simulink model "CF016A_GmVehSpdArbn"  (R2013b)
settings: Solver=FixedStepDiscrete  SolverMode=SingleTasking  StartTime=0.0  StopTime=1  FixedStep=0.002  RelTol=1e-3
undefined symbols (not defined in the file): DIAGCSTRTUPDLY_CNT_U32, NODEBSTEP_CNT_U16, NtcNr1, NtcSts1, VEHSPDMAX_KPH_F32
libraries: simulink x8, NxtrMax x7, NxtrMin x3, NxtrLim x3
(part 4 of 5)

== system CF016A_GmVehSpdArbn/GmVehSpdArbn/GmVehSpdArbnPer1/VehSpdMaxSecur_Invld ==
  Action Port : ActionPort  RequirementInfo="{'linktype_rmi_doors' '0000c6e6 (/GM T1XX/SubSystem Specifications/Customer Functions/CF016A GM Vehicle Speed Arbitration)' '#151' 'true' 'REQ:  151' '' } %GIDa_64e2156d_e885_4892_8ce8_3cf277fffe99"  ActionType=then
  Constant3 : Constant  RequirementInfo="{'linktype_rmi_doors' '0000c6e6 (/GM T1XX/SubSystem Specifications/Customer Functions/CF016A GM Vehicle Speed Arbitration)' '#151' 'true' 'REQ:  151' '' } %GIDa_7637d006_42b4_453b_9c6b_38d839e6b7ae"  Value=VEHSPDMAX_KPH_F32  OutDataTypeStr=single
      settings: AttributesFormatString=%<OutDataTypeStr>
  Constant4 : Constant  RequirementInfo="{'linktype_rmi_doors' '0000c6e6 (/GM T1XX/SubSystem Specifications/Customer Functions/CF016A GM Vehicle Speed Arbitration)' '#151' 'true' 'REQ:  151' '' } %GIDa_b234e855_697a_43ff_9746_9b343813ac54"  Value=false  OutDataTypeStr=boolean
      settings: AttributesFormatString=%<OutDataTypeStr>
  CopyRight2 : Subsystem  Description=|  RequirementInfo="{'linktype_rmi_doors' '0000c6e6 (/GM T1XX/SubSystem Specifications/Customer Functions/CF016A GM Vehicle Speed Arbitration)' '#151' 'true' 'REQ:  151' '' } %GIDa_55b8d56c_ea3d_4980_9cc8_0a4d021dc640"  mask(Copyright Information){none=on}
      | Copyright info block.                                               
      |                                                                     
      | Place copyright information at the top of every subsystem in design.
      mask prompts: none "No parameters"
      mask help: Place copyright information at the top of every subsystem in design.
      mask Display:
      | NxtrConf = 'Nexteer Confidential';
      | 
      | sys = bdroot; %handle for the current model ("system")
      | first = get_param(sys,'Created');
      | if(isempty(first))
      |     first = datestr(now,'yyyy');
      | else
      |     first = first(end-3:end);  %year is last four digits
      | end
      | 
      | last = get_param(sys,'LastModifiedDate');
      | if isempty(last)
      |     last = datestr(now,'yyyy');
      | else
      |     last = last(end-3:end);
      | end
      | 
      | if strcmp(first,last)
      |     fprintf('%s -- Copyright %s Nexteer',NxtrConf,first)
      | else
      |     fprintf('%s -- %s%s- %s Nexteer',NxtrConf,char(169),first,last)
      | end
  VehSpdMaxSecur : Outport  RequirementInfo="{'linktype_rmi_doors' '0000c6e6 (/GM T1XX/SubSystem Specifications/Customer Functions/CF016A GM Vehicle Speed Arbitration)' '#151' 'true' 'REQ:  151' '' } %GIDa_f81d9856_2c99_43a9_8580_21441ed5cbe9"
  VehSpdMaxSecurVld : Outport  RequirementInfo="{'linktype_rmi_doors' '0000c6e6 (/GM T1XX/SubSystem Specifications/Customer Functions/CF016A GM Vehicle Speed Arbitration)' '#151' 'true' 'REQ:  151' '' } %GIDa_72ce18ea_7958_4c7d_99d9_9239c29e1241"  Port=2
  wires:
  Constant3/1 -> VehSpdMaxSecur/1
  Constant4/1 -> VehSpdMaxSecurVld/1

== system CF016A_GmVehSpdArbn/GmVehSpdArbn/GmVehSpdArbnPer1/VehSpdMinSecur_Invld ==
  Action Port : ActionPort  ActionType=then
  Constant2 : Constant  RequirementInfo="{'linktype_rmi_doors' '0000c6e6 (/GM T1XX/SubSystem Specifications/Customer Functions/CF016A GM Vehicle Speed Arbitration)' '#200' 'true' 'REQ:  200' '' } %GIDa_8379dec2_765f_4e7e_be43_ecf0c6a82445"  Value=false  OutDataTypeStr=boolean
      settings: AttributesFormatString=%<OutDataTypeStr>
  Constant3 : Constant  RequirementInfo="{'linktype_rmi_doors' '0000c6e6 (/GM T1XX/SubSystem Specifications/Customer Functions/CF016A GM Vehicle Speed Arbitration)' '#200' 'true' 'REQ:  200' '' } %GIDa_805cec81_7588_4ea2_95e1_c6a565f2085e"  Value=0  OutDataTypeStr=single
      settings: AttributesFormatString=%<OutDataTypeStr>
  CopyRight2 : Subsystem  Description=|  mask(Copyright Information){none=on}
      | Copyright info block.                                               
      |                                                                     
      | Place copyright information at the top of every subsystem in design.
      mask prompts: none "No parameters"
      mask help: Place copyright information at the top of every subsystem in design.
      mask Display:
      | NxtrConf = 'Nexteer Confidential';
      | 
      | sys = bdroot; %handle for the current model ("system")
      | first = get_param(sys,'Created');
      | if(isempty(first))
      |     first = datestr(now,'yyyy');
      | else
      |     first = first(end-3:end);  %year is last four digits
      | end
      | 
      | last = get_param(sys,'LastModifiedDate');
      | if isempty(last)
      |     last = datestr(now,'yyyy');
      | else
      |     last = last(end-3:end);
      | end
      | 
      | if strcmp(first,last)
      |     fprintf('%s -- Copyright %s Nexteer',NxtrConf,first)
      | else
      |     fprintf('%s -- %s%s- %s Nexteer',NxtrConf,char(169),first,last)
      | end
  VehSpdMinSecur : Outport  RequirementInfo="{'linktype_rmi_doors' '0000c6e6 (/GM T1XX/SubSystem Specifications/Customer Functions/CF016A GM Vehicle Speed Arbitration)' '#200' 'true' 'REQ:  200' '' } %GIDa_4848a70f_3ce8_4b37_84fd_cdad733c9f51"
  VehSpdMinSecurVld : Outport  RequirementInfo="{'linktype_rmi_doors' '0000c6e6 (/GM T1XX/SubSystem Specifications/Customer Functions/CF016A GM Vehicle Speed Arbitration)' '#200' 'true' 'REQ:  200' '' } %GIDa_aef7dbb3_b6b0_484d_bb99_ef1c2a4a1cac"  Port=2
  wires:
  Constant2/1 -> VehSpdMinSecurVld/1
  Constant3/1 -> VehSpdMinSecur/1

== system CF016A_GmVehSpdArbn/GmVehSpdArbn/GmVehSpdArbnInit1/GetRefTmr100MicroSec32bit/CopyRight2 ==

== system CF016A_GmVehSpdArbn/GmVehSpdArbn/GmVehSpdArbnPer1/ArbdFalseAndSnsrFalse_NTCFaild/CopyRight2 ==

== system CF016A_GmVehSpdArbn/GmVehSpdArbn/GmVehSpdArbnPer1/ArbdFalseAndSnsrFalse_NTCFaild/NTC_0x0E0 ==
  NtcNr : Inport
  NtcStInfo : Inport  Port=2
  NtcSts : Inport  Port=3
  DebStep : Inport  Port=4
  CallDiagMgr : ActionPort  ActionType=then
  SetNtcSts : Subsystem  RequirementInfo={} %GIDa_9ed89afc_c0fd_408c_a804_1b2e1348b82a  TreatAsAtomicUnit=on
      settings: RTWSystemCode=Inline
  wires:
  NtcNr/1 -> SetNtcSts/1(NtcNr)  "NtcNr"
  NtcSts/1 -> SetNtcSts/3(NtcSts)
  DebStep/1 -> SetNtcSts/4(DebStep)
  NtcStInfo/1 -> SetNtcSts/2(NtcStInfo)

== system CF016A_GmVehSpdArbn/GmVehSpdArbn/GmVehSpdArbnPer1/ArbdFalseAndSnsrTrue_NTCPassd/CopyRight2 ==

== system CF016A_GmVehSpdArbn/GmVehSpdArbn/GmVehSpdArbnPer1/ArbdFalseAndSnsrTrue_NTCPassd/NTC_0x0E0 ==
  NtcNr : Inport
  NtcStInfo : Inport  Port=2
  NtcSts : Inport  Port=3
  DebStep : Inport  Port=4
  CallDiagMgr : ActionPort  ActionType=then
  SetNtcSts : Subsystem  RequirementInfo={} %GIDa_edd408d1_9bb5_4017_8804_a8b180852b3e  TreatAsAtomicUnit=on
      settings: RTWSystemCode=Inline
  wires:
  NtcStInfo/1 -> SetNtcSts/2(NtcStInfo)
  DebStep/1 -> SetNtcSts/4(DebStep)
  NtcSts/1 -> SetNtcSts/3(NtcSts)
  NtcNr/1 -> SetNtcSts/1(NtcNr)  "NtcNr"

== system CF016A_GmVehSpdArbn/GmVehSpdArbn/GmVehSpdArbnPer1/ArbdTrueAndSnsrTrue_NTCPassd/CopyRight2 ==

== system CF016A_GmVehSpdArbn/GmVehSpdArbn/GmVehSpdArbnPer1/ArbdTrueAndSnsrTrue_NTCPassd/NTC_0x0E0 ==
  NtcNr : Inport
  NtcStInfo : Inport  Port=2
  NtcSts : Inport  Port=3
  DebStep : Inport  Port=4
  CallDiagMgr : ActionPort  ActionType=then
  SetNtcSts : Subsystem  RequirementInfo={} %GIDa_c0105d74_7713_458a_af4f_14b36b448539  TreatAsAtomicUnit=on
      settings: RTWSystemCode=Inline
  wires:
  NtcStInfo/1 -> SetNtcSts/2(NtcStInfo)
  DebStep/1 -> SetNtcSts/4(DebStep)
  NtcSts/1 -> SetNtcSts/3(NtcSts)
  NtcNr/1 -> SetNtcSts/1(NtcNr)  "NtcNr"

== system CF016A_GmVehSpdArbn/GmVehSpdArbn/GmVehSpdArbnPer1/Calc_NTCIdleTi/CopyRight2 ==

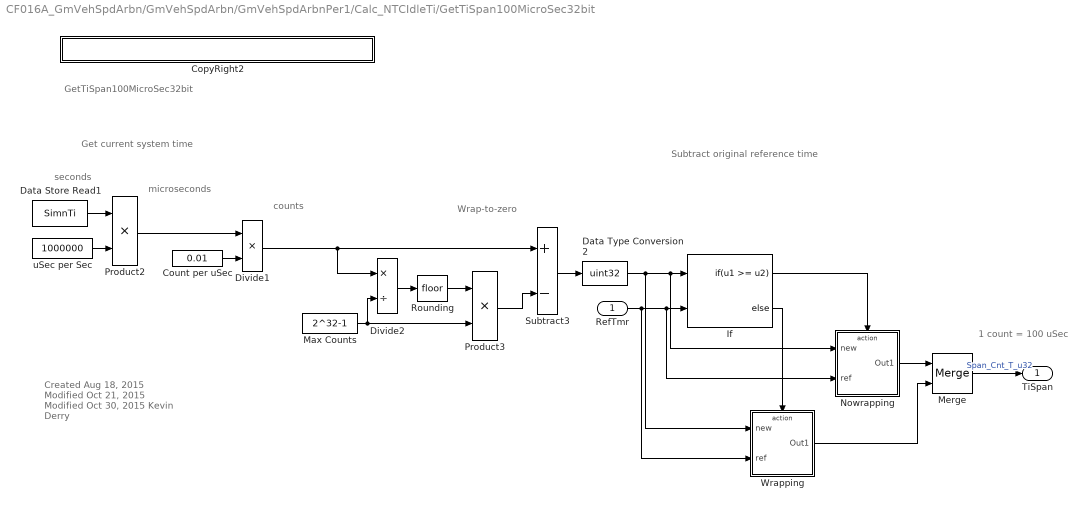
== system CF016A_GmVehSpdArbn/GmVehSpdArbn/GmVehSpdArbnPer1/Calc_NTCIdleTi/GetTiSpan100MicroSec32bit ==
  note: Created Aug 18, 2015
      | Modified Oct 21, 2015
      | Modified Oct 30, 2015
      | Kevin Derry
  note: GetTiSpan100MicroSec32bit
  note: Get current system time
  note: 1 count = 100 uSec
  note: Wrap-to-zero
  note: counts
  note: microseconds
  note: seconds
  note: Subtract original reference time
  RefTmr : Inport
  CopyRight2 : Subsystem  Description=|  mask(Copyright Information){none=on}
      | Copyright info block.                                               
      |                                                                     
      | Place copyright information at the top of every subsystem in design.
      mask prompts: none "No parameters"
      mask help: Place copyright information at the top of every subsystem in design.
      mask Display:
      | NxtrConf = 'Nexteer Confidential';
      | 
      | sys = bdroot; %handle for the current model ("system")
      | first = get_param(sys,'Created');
      | if(isempty(first))
      |     first = datestr(now,'yyyy');
      | else
      |     first = first(end-3:end);  %year is last four digits
      | end
      | 
      | last = get_param(sys,'LastModifiedDate');
      | if isempty(last)
      |     last = datestr(now,'yyyy');
      | else
      |     last = last(end-3:end);
      | end
      | 
      | if strcmp(first,last)
      |     fprintf('%s -- Copyright %s Nexteer',NxtrConf,first)
      | else
      |     fprintf('%s -- %s%s- %s Nexteer',NxtrConf,char(169),first,last)
      | end
  Count per uSec : Constant  Value=0.01
  Data Store Read1 : DataStoreRead  DataStoreName=SimnTi
  Data Type Conversion2 : DataTypeConversion  OutDataTypeStr=uint32
  Divide1 : Product  Inputs=**
  Divide2 : Product  Inputs=*/
  If : If  NumInputs=2  IfExpression=u1 >= u2
  Max Counts : Constant  Value=2^32-1
  Merge : Merge
  Nowrapping : Subsystem  TreatAsAtomicUnit=on
  Product2 : Product
  Product3 : Product
  Rounding : Rounding
  Subtract3 : Sum  Inputs=+-
  Wrapping : Subsystem  TreatAsAtomicUnit=on
  uSec per Sec : Constant  Value=1000000
  TiSpan : Outport
  wires:
  Data Type Conversion2/1 -> Wrapping/1(new), Nowrapping/1(new), If/1
  RefTmr/1 -> Wrapping/2(ref), Nowrapping/2(ref), If/2
  Merge/1 -> TiSpan/1  "Span_Cnt_T_u32"
  uSec per Sec/1 -> Product2/2
  Count per uSec/1 -> Divide1/2
  Data Store Read1/1 -> Product2/1
  Product2/1 -> Divide1/1
  Divide1/1 -> Subtract3/1, Divide2/1
  Max Counts/1 -> Product3/2, Divide2/2
  Divide2/1 -> Rounding/1
  Rounding/1 -> Product3/1
  Subtract3/1 -> Data Type Conversion2/1
  Product3/1 -> Subtract3/2
  If/1 -> Nowrapping/Action
  If/2 -> Wrapping/Action
  Nowrapping/1(Out1) -> Merge/1
  Wrapping/1(Out1) -> Merge/2

== system CF016A_GmVehSpdArbn/GmVehSpdArbn/GmVehSpdArbnPer1/Calc_SpdArbd/Calc_VehSpdArbd ==
  TmpSpdArbd : Inport  RequirementInfo={} %GIDa_22ee0604_b96b_41df_b3cf_508af8afbd88
  TmpSpdArbdCnt : Inport  RequirementInfo={} %GIDa_d3815bce_edc7_4bfa_b1ce_5bf581d265aa  Port=2
  Action Port : ActionPort  ActionType=then
  CopyRight2 : Subsystem  Description=|  mask(Copyright Information){none=on}
      | Copyright info block.                                               
      |                                                                     
      | Place copyright information at the top of every subsystem in design.
      mask prompts: none "No parameters"
      mask help: Place copyright information at the top of every subsystem in design.
      mask Display:
      | NxtrConf = 'Nexteer Confidential';
      | 
      | sys = bdroot; %handle for the current model ("system")
      | first = get_param(sys,'Created');
      | if(isempty(first))
      |     first = datestr(now,'yyyy');
      | else
      |     first = first(end-3:end);  %year is last four digits
      | end
      | 
      | last = get_param(sys,'LastModifiedDate');
      | if isempty(last)
      |     last = datestr(now,'yyyy');
      | else
      |     last = last(end-3:end);
      | end
      | 
      | if strcmp(first,last)
      |     fprintf('%s -- Copyright %s Nexteer',NxtrConf,first)
      | else
      |     fprintf('%s -- %s%s- %s Nexteer',NxtrConf,char(169),first,last)
      | end
  Divide : Product  Inputs=*/
  SpdArbd : Outport
  wires:
  TmpSpdArbd/1 -> Divide/1
  TmpSpdArbdCnt/1 -> Divide/2
  Divide/1 -> SpdArbd/1

== system CF016A_GmVehSpdArbn/GmVehSpdArbn/GmVehSpdArbnPer1/Calc_SpdArbd/CopyRight2 ==

== system CF016A_GmVehSpdArbn/GmVehSpdArbn/GmVehSpdArbnPer1/Calc_SpdArbd/Pass_TmpSpdArbd ==
  TmpSpdArbd : Inport  RequirementInfo={} %GIDa_a9ccc6d1_62c5_46ea_817b_212a243cba27
  Action Port : ActionPort  ActionType=else
  CopyRight2 : Subsystem  Description=|  mask(Copyright Information){none=on}
      | Copyright info block.                                               
      |                                                                     
      | Place copyright information at the top of every subsystem in design.
      mask prompts: none "No parameters"
      mask help: Place copyright information at the top of every subsystem in design.
      mask Display:
      | NxtrConf = 'Nexteer Confidential';
      | 
      | sys = bdroot; %handle for the current model ("system")
      | first = get_param(sys,'Created');
      | if(isempty(first))
      |     first = datestr(now,'yyyy');
      | else
      |     first = first(end-3:end);  %year is last four digits
      | end
      | 
      | last = get_param(sys,'LastModifiedDate');
      | if isempty(last)
      |     last = datestr(now,'yyyy');
      | else
      |     last = last(end-3:end);
      | end
      | 
      | if strcmp(first,last)
      |     fprintf('%s -- Copyright %s Nexteer',NxtrConf,first)
      | else
      |     fprintf('%s -- %s%s- %s Nexteer',NxtrConf,char(169),first,last)
      | end
  VehSpdArbd : Outport
  wires:
  TmpSpdArbd/1 -> VehSpdArbd/1

== system CF016A_GmVehSpdArbn/GmVehSpdArbn/GmVehSpdArbnPer1/Calc_TmpSpdArbd_SpdArbdCnt/CalcSumCnt ==
  TmpSpdIn : Inport  RequirementInfo={} %GIDa_cc3fdd2f_e00a_4d73_ad47_b131220ca799
  RiDrvnBusHiSpd : Inport  RequirementInfo={} %GIDa_bdf168f4_a9f1_4976_b82a_f5282d73e040  Port=2
  CntIn : Inport  RequirementInfo={} %GIDa_335889c6_d315_49b5_8e0c_287140eef7c6  Port=3
  Action Port : ActionPort  ActionType=then
  Add : Sum
  Add1 : Sum
  Constant2 : Constant  OutDataTypeStr=single
      settings: AttributesFormatString=%<OutDataTypeStr>
  CopyRight2 : Subsystem  Description=|  mask(Copyright Information){none=on}
      | Copyright info block.                                               
      |                                                                     
      | Place copyright information at the top of every subsystem in design.
      mask prompts: none "No parameters"
      mask help: Place copyright information at the top of every subsystem in design.
      mask Display:
      | NxtrConf = 'Nexteer Confidential';
      | 
      | sys = bdroot; %handle for the current model ("system")
      | first = get_param(sys,'Created');
      | if(isempty(first))
      |     first = datestr(now,'yyyy');
      | else
      |     first = first(end-3:end);  %year is last four digits
      | end
      | 
      | last = get_param(sys,'LastModifiedDate');
      | if isempty(last)
      |     last = datestr(now,'yyyy');
      | else
      |     last = last(end-3:end);
      | end
      | 
      | if strcmp(first,last)
      |     fprintf('%s -- Copyright %s Nexteer',NxtrConf,first)
      | else
      |     fprintf('%s -- %s%s- %s Nexteer',NxtrConf,char(169),first,last)
      | end
  TmpSpdArbd : Outport
  SpdArbdCnt : Outport  Port=2
  wires:
  Add1/1 -> SpdArbdCnt/1
  Constant2/1 -> Add1/2
  CntIn/1 -> Add1/1
  TmpSpdIn/1 -> Add/2
  RiDrvnBusHiSpd/1 -> Add/1
  Add/1 -> TmpSpdArbd/1

== system CF016A_GmVehSpdArbn/GmVehSpdArbn/GmVehSpdArbnPer1/Calc_TmpSpdArbd_SpdArbdCnt/CalcSumCnt_1 ==
  LeNonDrvnBusHiSpd : Inport  RequirementInfo={} %GIDa_850f1153_ec6b_472c_bf3f_b4555508d628
  TmpSpdIn : Inport  RequirementInfo={} %GIDa_8bdfcdcf_300c_498e_8ae0_3709bc028ab2  Port=2
  CntIn : Inport  RequirementInfo={} %GIDa_524e2e91_4b78_4f70_98dc_26836a52cb3a  Port=3
  Action Port : ActionPort  ActionType=then
  Add : Sum
  Add1 : Sum
  Constant2 : Constant  OutDataTypeStr=single
      settings: AttributesFormatString=%<OutDataTypeStr>
  CopyRight2 : Subsystem  Description=|  mask(Copyright Information){none=on}
      | Copyright info block.                                               
      |                                                                     
      | Place copyright information at the top of every subsystem in design.
      mask prompts: none "No parameters"
      mask help: Place copyright information at the top of every subsystem in design.
      mask Display:
      | NxtrConf = 'Nexteer Confidential';
      | 
      | sys = bdroot; %handle for the current model ("system")
      | first = get_param(sys,'Created');
      | if(isempty(first))
      |     first = datestr(now,'yyyy');
      | else
      |     first = first(end-3:end);  %year is last four digits
      | end
      | 
      | last = get_param(sys,'LastModifiedDate');
      | if isempty(last)
      |     last = datestr(now,'yyyy');
      | else
      |     last = last(end-3:end);
      | end
      | 
      | if strcmp(first,last)
      |     fprintf('%s -- Copyright %s Nexteer',NxtrConf,first)
      | else
      |     fprintf('%s -- %s%s- %s Nexteer',NxtrConf,char(169),first,last)
      | end
  TmpSpdArbd : Outport
  SpdArbdCnt : Outport  Port=2
  wires:
  Add/1 -> TmpSpdArbd/1
  TmpSpdIn/1 -> Add/1
  LeNonDrvnBusHiSpd/1 -> Add/2
  CntIn/1 -> Add1/1
  Constant2/1 -> Add1/2
  Add1/1 -> SpdArbdCnt/1

== system CF016A_GmVehSpdArbn/GmVehSpdArbn/GmVehSpdArbnPer1/Calc_TmpSpdArbd_SpdArbdCnt/CalcSumCnt_2 ==
  TmpSpdIn : Inport  RequirementInfo={} %GIDa_8e0c55ff_68c1_41a4_a413_79990270a578
  RiNonDrvnBusHiSpd : Inport  RequirementInfo={} %GIDa_75592bc1_7625_4699_8c9b_f1eb2e030f50  Port=2
  CntIn : Inport  RequirementInfo={} %GIDa_c479272c_0732_4e1a_8e5e_d31eed4afd4e  Port=3
  Action Port : ActionPort  ActionType=then
  Add : Sum
  Add1 : Sum
  Constant2 : Constant  OutDataTypeStr=single
      settings: AttributesFormatString=%<OutDataTypeStr>
  CopyRight2 : Subsystem  Description=|  mask(Copyright Information){none=on}
      | Copyright info block.                                               
      |                                                                     
      | Place copyright information at the top of every subsystem in design.
      mask prompts: none "No parameters"
      mask help: Place copyright information at the top of every subsystem in design.
      mask Display:
      | NxtrConf = 'Nexteer Confidential';
      | 
      | sys = bdroot; %handle for the current model ("system")
      | first = get_param(sys,'Created');
      | if(isempty(first))
      |     first = datestr(now,'yyyy');
      | else
      |     first = first(end-3:end);  %year is last four digits
      | end
      | 
      | last = get_param(sys,'LastModifiedDate');
      | if isempty(last)
      |     last = datestr(now,'yyyy');
      | else
      |     last = last(end-3:end);
      | end
      | 
      | if strcmp(first,last)
      |     fprintf('%s -- Copyright %s Nexteer',NxtrConf,first)
      | else
      |     fprintf('%s -- %s%s- %s Nexteer',NxtrConf,char(169),first,last)
      | end
  TmpSpdArbd : Outport
  SpdArbdCnt : Outport  Port=2
  wires:
  Add1/1 -> SpdArbdCnt/1
  Constant2/1 -> Add1/2
  CntIn/1 -> Add1/1
  TmpSpdIn/1 -> Add/2
  RiNonDrvnBusHiSpd/1 -> Add/1
  Add/1 -> TmpSpdArbd/1

== system CF016A_GmVehSpdArbn/GmVehSpdArbn/GmVehSpdArbnPer1/Calc_TmpSpdArbd_SpdArbdCnt/CalcSumCnt_3 ==
  TmpSpdIn : Inport  RequirementInfo={} %GIDa_27ed8032_b8a3_44e7_a82c_716af4549a85
  LeDrvnBusHiSpd : Inport  RequirementInfo={} %GIDa_c96c6b2e_7259_40ac_8462_8989bfe94a44  Port=2
  CntIn : Inport  RequirementInfo={} %GIDa_dfbf4464_a6c1_42ad_8ec2_154e9928d5a6  Port=3
  Action Port : ActionPort  ActionType=then
  Add : Sum
  Add1 : Sum
  Constant2 : Constant  OutDataTypeStr=single
      settings: AttributesFormatString=%<OutDataTypeStr>
  CopyRight2 : Subsystem  Description=|  mask(Copyright Information){none=on}
      | Copyright info block.                                               
      |                                                                     
      | Place copyright information at the top of every subsystem in design.
      mask prompts: none "No parameters"
      mask help: Place copyright information at the top of every subsystem in design.
      mask Display:
      | NxtrConf = 'Nexteer Confidential';
      | 
      | sys = bdroot; %handle for the current model ("system")
      | first = get_param(sys,'Created');
      | if(isempty(first))
      |     first = datestr(now,'yyyy');
      | else
      |     first = first(end-3:end);  %year is last four digits
      | end
      | 
      | last = get_param(sys,'LastModifiedDate');
      | if isempty(last)
      |     last = datestr(now,'yyyy');
      | else
      |     last = last(end-3:end);
      | end
      | 
      | if strcmp(first,last)
      |     fprintf('%s -- Copyright %s Nexteer',NxtrConf,first)
      | else
      |     fprintf('%s -- %s%s- %s Nexteer',NxtrConf,char(169),first,last)
      | end
  TmpSpdArbd : Outport
  SpdArbdCnt : Outport  Port=2
  wires:
  Add/1 -> TmpSpdArbd/1
  LeDrvnBusHiSpd/1 -> Add/1
  TmpSpdIn/1 -> Add/2
  CntIn/1 -> Add1/1
  Constant2/1 -> Add1/2
  Add1/1 -> SpdArbdCnt/1

== system CF016A_GmVehSpdArbn/GmVehSpdArbn/GmVehSpdArbnPer1/Calc_TmpSpdArbd_SpdArbdCnt/CopyRight2 ==

== system CF016A_GmVehSpdArbn/GmVehSpdArbn/GmVehSpdArbnPer1/Calc_TmpSpdArbd_SpdArbdCnt/Pass_0s ==
  TmpSpdIn : Inport  RequirementInfo={} %GIDa_c245ec3d_ac7f_433e_a7eb_117742686023
  CntIn : Inport  RequirementInfo={} %GIDa_04336cb5_f5d6_482b_a7a3_24a26aa66881  Port=2
  Action Port : ActionPort  ActionType=else
  CopyRight2 : Subsystem  Description=|  mask(Copyright Information){none=on}
      | Copyright info block.                                               
      |                                                                     
      | Place copyright information at the top of every subsystem in design.
      mask prompts: none "No parameters"
      mask help: Place copyright information at the top of every subsystem in design.
      mask Display:
      | NxtrConf = 'Nexteer Confidential';
      | 
      | sys = bdroot; %handle for the current model ("system")
      | first = get_param(sys,'Created');
      | if(isempty(first))
      |     first = datestr(now,'yyyy');
      | else
      |     first = first(end-3:end);  %year is last four digits
      | end
      | 
      | last = get_param(sys,'LastModifiedDate');
      | if isempty(last)
      |     last = datestr(now,'yyyy');
      | else
      |     last = last(end-3:end);
      | end
      | 
      | if strcmp(first,last)
      |     fprintf('%s -- Copyright %s Nexteer',NxtrConf,first)
      | else
      |     fprintf('%s -- %s%s- %s Nexteer',NxtrConf,char(169),first,last)
      | end
  TmpSpdArbd : Outport
  SpdArbdCnt : Outport  Port=2
  wires:
  CntIn/1 -> SpdArbdCnt/1
  TmpSpdIn/1 -> TmpSpdArbd/1

== system CF016A_GmVehSpdArbn/GmVehSpdArbn/GmVehSpdArbnPer1/Calc_TmpSpdArbd_SpdArbdCnt/Pass_TmpSpdArbd_SpdArbdCnt_1 ==
  TmpSpdIn : Inport  RequirementInfo={} %GIDa_be392035_672d_4555_8348_f6cb397ff1c2
  CntIn : Inport  RequirementInfo={} %GIDa_b54fbdf8_af01_4bd7_a959_8ca2986c3520  Port=2
  Action Port : ActionPort  ActionType=else
  CopyRight2 : Subsystem  Description=|  mask(Copyright Information){none=on}
      | Copyright info block.                                               
      |                                                                     
      | Place copyright information at the top of every subsystem in design.
      mask prompts: none "No parameters"
      mask help: Place copyright information at the top of every subsystem in design.
      mask Display:
      | NxtrConf = 'Nexteer Confidential';
      | 
      | sys = bdroot; %handle for the current model ("system")
      | first = get_param(sys,'Created');
      | if(isempty(first))
      |     first = datestr(now,'yyyy');
      | else
      |     first = first(end-3:end);  %year is last four digits
      | end
      | 
      | last = get_param(sys,'LastModifiedDate');
      | if isempty(last)
      |     last = datestr(now,'yyyy');
      | else
      |     last = last(end-3:end);
      | end
      | 
      | if strcmp(first,last)
      |     fprintf('%s -- Copyright %s Nexteer',NxtrConf,first)
      | else
      |     fprintf('%s -- %s%s- %s Nexteer',NxtrConf,char(169),first,last)
      | end
  TmpSpdArbd : Outport
  SpdArbdCnt : Outport  Port=2
  wires:
  CntIn/1 -> SpdArbdCnt/1
  TmpSpdIn/1 -> TmpSpdArbd/1

== system CF016A_GmVehSpdArbn/GmVehSpdArbn/GmVehSpdArbnPer1/Calc_TmpSpdArbd_SpdArbdCnt/Pass_TmpSpdArbd_SpdArbdCnt_2 ==
  TmpSpdIn : Inport  RequirementInfo={} %GIDa_c2285e44_32b2_4691_a335_e8a509434fe3
  CntIn : Inport  RequirementInfo={} %GIDa_b6863996_5c43_4ec4_8339_06ddcee963ca  Port=2
  Action Port : ActionPort  ActionType=else
  CopyRight2 : Subsystem  Description=|  mask(Copyright Information){none=on}
      | Copyright info block.                                               
      |                                                                     
      | Place copyright information at the top of every subsystem in design.
      mask prompts: none "No parameters"
      mask help: Place copyright information at the top of every subsystem in design.
      mask Display:
      | NxtrConf = 'Nexteer Confidential';
      | 
      | sys = bdroot; %handle for the current model ("system")
      | first = get_param(sys,'Created');
      | if(isempty(first))
      |     first = datestr(now,'yyyy');
      | else
      |     first = first(end-3:end);  %year is last four digits
      | end
      | 
      | last = get_param(sys,'LastModifiedDate');
      | if isempty(last)
      |     last = datestr(now,'yyyy');
      | else
      |     last = last(end-3:end);
      | end
      | 
      | if strcmp(first,last)
      |     fprintf('%s -- Copyright %s Nexteer',NxtrConf,first)
      | else
      |     fprintf('%s -- %s%s- %s Nexteer',NxtrConf,char(169),first,last)
      | end
  TmpSpdArbd : Outport
  SpdArbdCnt : Outport  Port=2
  wires:
  TmpSpdIn/1 -> TmpSpdArbd/1
  CntIn/1 -> SpdArbdCnt/1

== system CF016A_GmVehSpdArbn/GmVehSpdArbn/GmVehSpdArbnPer1/Calc_TmpSpdArbd_SpdArbdCnt/Pass_TmpSpdArbd_SpdArbdCnt_3 ==
  TmpSpdIn : Inport  RequirementInfo={} %GIDa_5e5df1f6_8ff4_4858_9989_4bafd778ca0f
  CntIn : Inport  RequirementInfo={} %GIDa_0592b7e3_be9b_4836_9a53_c8b365bd076c  Port=2
  Action Port : ActionPort  ActionType=else
  CopyRight2 : Subsystem  Description=|  mask(Copyright Information){none=on}
      | Copyright info block.                                               
      |                                                                     
      | Place copyright information at the top of every subsystem in design.
      mask prompts: none "No parameters"
      mask help: Place copyright information at the top of every subsystem in design.
      mask Display:
      | NxtrConf = 'Nexteer Confidential';
      | 
      | sys = bdroot; %handle for the current model ("system")
      | first = get_param(sys,'Created');
      | if(isempty(first))
      |     first = datestr(now,'yyyy');
      | else
      |     first = first(end-3:end);  %year is last four digits
      | end
      | 
      | last = get_param(sys,'LastModifiedDate');
      | if isempty(last)
      |     last = datestr(now,'yyyy');
      | else
      |     last = last(end-3:end);
      | end
      | 
      | if strcmp(first,last)
      |     fprintf('%s -- Copyright %s Nexteer',NxtrConf,first)
      | else
      |     fprintf('%s -- %s%s- %s Nexteer',NxtrConf,char(169),first,last)
      | end
  TmpSpdArbd : Outport
  SpdArbdCnt : Outport  Port=2
  wires:
  CntIn/1 -> SpdArbdCnt/1
  TmpSpdIn/1 -> TmpSpdArbd/1

== system CF016A_GmVehSpdArbn/GmVehSpdArbn/GmVehSpdArbnPer1/Calc_VehSpdMaxSecur/Calc_VehSpdMaxSecur ==
  VehSpdMaxSecur : Inport  RequirementInfo={} %GIDa_b1037a0f_d275_40dd_a845_e9fde032183c
  WhlGndVelRiNonDrvnBusChassisExp : Inport  RequirementInfo={} %GIDa_398e957f_9e7e_45fc_917b_0fc3d04e1e46  Port=2
  WhlGndVelRiNonDrvnBusHiSpd : Inport  RequirementInfo={} %GIDa_085660d0_509a_4113_872b_79769319dc23  Port=3
  Action Port : ActionPort  ActionType=then
  CopyRight2 : Subsystem  Description=|  mask(Copyright Information){none=on}
      | Copyright info block.                                               
      |                                                                     
      | Place copyright information at the top of every subsystem in design.
      mask prompts: none "No parameters"
      mask help: Place copyright information at the top of every subsystem in design.
      mask Display:
      | NxtrConf = 'Nexteer Confidential';
      | 
      | sys = bdroot; %handle for the current model ("system")
      | first = get_param(sys,'Created');
      | if(isempty(first))
      |     first = datestr(now,'yyyy');
      | else
      |     first = first(end-3:end);  %year is last four digits
      | end
      | 
      | last = get_param(sys,'LastModifiedDate');
      | if isempty(last)
      |     last = datestr(now,'yyyy');
      | else
      |     last = last(end-3:end);
      | end
      | 
      | if strcmp(first,last)
      |     fprintf('%s -- Copyright %s Nexteer',NxtrConf,first)
      | else
      |     fprintf('%s -- %s%s- %s Nexteer',NxtrConf,char(169),first,last)
      | end
  Max_f1 : NxtrMax/Max_f32  SFunctionSpec=single y1 = Max_f32(single u1, single u2)
      settings: AttributesFormatString=%<Name>
  Max_f32 : NxtrMax/Max_f32  SFunctionSpec=single y1 = Max_f32(single u1, single u2)
      settings: AttributesFormatString=%<Name>
  TmpVehSpdMaxSecur : Outport
  wires:
  Max_f1/1 -> TmpVehSpdMaxSecur/1
  Max_f32/1 -> Max_f1/1
  VehSpdMaxSecur/1 -> Max_f32/1
  WhlGndVelRiNonDrvnBusChassisExp/1 -> Max_f32/2
  WhlGndVelRiNonDrvnBusHiSpd/1 -> Max_f1/2

== system CF016A_GmVehSpdArbn/GmVehSpdArbn/GmVehSpdArbnPer1/Calc_VehSpdMaxSecur/Calc_VehSpdMaxSecur1 ==
  WhlGndVelLeDrvnBusChassisExp : Inport  RequirementInfo={} %GIDa_a5714172_ef06_41ef_b8c5_c003cd29fe6a  OutDataTypeStr=single
  WhlGndVelLeDrvnBusHiSpd : Inport  RequirementInfo={} %GIDa_0d911216_cd59_4389_bf95_6fb3bce5f572  Port=2
  Action Port : ActionPort  ActionType=then
  CopyRight2 : Subsystem  Description=|  mask(Copyright Information){none=on}
      | Copyright info block.                                               
      |                                                                     
      | Place copyright information at the top of every subsystem in design.
      mask prompts: none "No parameters"
      mask help: Place copyright information at the top of every subsystem in design.
      mask Display:
      | NxtrConf = 'Nexteer Confidential';
      | 
      | sys = bdroot; %handle for the current model ("system")
      | first = get_param(sys,'Created');
      | if(isempty(first))
      |     first = datestr(now,'yyyy');
      | else
      |     first = first(end-3:end);  %year is last four digits
      | end
      | 
      | last = get_param(sys,'LastModifiedDate');
      | if isempty(last)
      |     last = datestr(now,'yyyy');
      | else
      |     last = last(end-3:end);
      | end
      | 
      | if strcmp(first,last)
      |     fprintf('%s -- Copyright %s Nexteer',NxtrConf,first)
      | else
      |     fprintf('%s -- %s%s- %s Nexteer',NxtrConf,char(169),first,last)
      | end
  Max_f1 : NxtrMax/Max_f32  SFunctionSpec=single y1 = Max_f32(single u1, single u2)
      settings: AttributesFormatString=%<Name>
  TmpVehSpdMaxSecur : Outport
  wires:
  WhlGndVelLeDrvnBusChassisExp/1 -> Max_f1/1
  WhlGndVelLeDrvnBusHiSpd/1 -> Max_f1/2
  Max_f1/1 -> TmpVehSpdMaxSecur/1

== system CF016A_GmVehSpdArbn/GmVehSpdArbn/GmVehSpdArbnPer1/Calc_VehSpdMaxSecur/Calc_VehSpdMaxSecur2 ==
  VehSpdMaxSecur : Inport  RequirementInfo={} %GIDa_fb4a03b7_59b8_42b9_ae90_c80297cd9f02
  WhlGndVelRiDrvnBusChassisExp : Inport  RequirementInfo={} %GIDa_102b8552_b00d_4cd9_9963_710886a19734  Port=2
  WhlGndVelRiDrvnBusHiSpd : Inport  RequirementInfo={} %GIDa_b2136e85_a696_434d_9517_6bcdf82f8f4e  Port=3
  Action Port : ActionPort  ActionType=then
  CopyRight2 : Subsystem  Description=|  mask(Copyright Information){none=on}
      | Copyright info block.                                               
      |                                                                     
      | Place copyright information at the top of every subsystem in design.
      mask prompts: none "No parameters"
      mask help: Place copyright information at the top of every subsystem in design.
      mask Display:
      | NxtrConf = 'Nexteer Confidential';
      | 
      | sys = bdroot; %handle for the current model ("system")
      | first = get_param(sys,'Created');
      | if(isempty(first))
      |     first = datestr(now,'yyyy');
      | else
      |     first = first(end-3:end);  %year is last four digits
      | end
      | 
      | last = get_param(sys,'LastModifiedDate');
      | if isempty(last)
      |     last = datestr(now,'yyyy');
      | else
      |     last = last(end-3:end);
      | end
      | 
      | if strcmp(first,last)
      |     fprintf('%s -- Copyright %s Nexteer',NxtrConf,first)
      | else
      |     fprintf('%s -- %s%s- %s Nexteer',NxtrConf,char(169),first,last)
      | end
  Max_f1 : NxtrMax/Max_f32  SFunctionSpec=single y1 = Max_f32(single u1, single u2)
      settings: AttributesFormatString=%<Name>
  Max_f32 : NxtrMax/Max_f32  SFunctionSpec=single y1 = Max_f32(single u1, single u2)
      settings: AttributesFormatString=%<Name>
  TmpVehSpdMaxSecur : Outport
  wires:
  Max_f1/1 -> TmpVehSpdMaxSecur/1
  WhlGndVelRiDrvnBusHiSpd/1 -> Max_f1/2
  Max_f32/1 -> Max_f1/1
  VehSpdMaxSecur/1 -> Max_f32/1
  WhlGndVelRiDrvnBusChassisExp/1 -> Max_f32/2

== system CF016A_GmVehSpdArbn/GmVehSpdArbn/GmVehSpdArbnPer1/Calc_VehSpdMaxSecur/Calc_VehSpdMaxSecur3 ==
  VehSpdMaxSecur : Inport  RequirementInfo={} %GIDa_64646bcd_c362_464f_8cf7_4188f80b1217
  WhlGndVelLeNonDrvnBusHiSpd : Inport  RequirementInfo={} %GIDa_65d4786b_189d_45bd_970b_8c10ca946198  Port=2
  WhlGndVelLeNonDrvnBusChassisExp : Inport  RequirementInfo={} %GIDa_a4bb593a_97fb_4b76_9b54_13fc6dfedc76  Port=3
  Action Port : ActionPort  ActionType=then
  CopyRight2 : Subsystem  Description=|  mask(Copyright Information){none=on}
      | Copyright info block.                                               
      |                                                                     
      | Place copyright information at the top of every subsystem in design.
      mask prompts: none "No parameters"
      mask help: Place copyright information at the top of every subsystem in design.
      mask Display:
      | NxtrConf = 'Nexteer Confidential';
      | 
      | sys = bdroot; %handle for the current model ("system")
      | first = get_param(sys,'Created');
      | if(isempty(first))
      |     first = datestr(now,'yyyy');
      | else
      |     first = first(end-3:end);  %year is last four digits
      | end
      | 
      | last = get_param(sys,'LastModifiedDate');
      | if isempty(last)
      |     last = datestr(now,'yyyy');
      | else
      |     last = last(end-3:end);
      | end
      | 
      | if strcmp(first,last)
      |     fprintf('%s -- Copyright %s Nexteer',NxtrConf,first)
      | else
      |     fprintf('%s -- %s%s- %s Nexteer',NxtrConf,char(169),first,last)
      | end
  Max_f1 : NxtrMax/Max_f32  SFunctionSpec=single y1 = Max_f32(single u1, single u2)
      settings: AttributesFormatString=%<Name>
  Max_f32 : NxtrMax/Max_f32  SFunctionSpec=single y1 = Max_f32(single u1, single u2)
      settings: AttributesFormatString=%<Name>
  TmpVehSpdMaxSecur : Outport
  wires:
  WhlGndVelLeNonDrvnBusHiSpd/1 -> Max_f32/2
  VehSpdMaxSecur/1 -> Max_f32/1
  Max_f32/1 -> Max_f1/1
  WhlGndVelLeNonDrvnBusChassisExp/1 -> Max_f1/2
  Max_f1/1 -> TmpVehSpdMaxSecur/1

== system CF016A_GmVehSpdArbn/GmVehSpdArbn/GmVehSpdArbnPer1/Calc_VehSpdMaxSecur/CopyRight2 ==

== system CF016A_GmVehSpdArbn/GmVehSpdArbn/GmVehSpdArbnPer1/Calc_VehSpdMaxSecur/Pass_0 ==
  VehSpdMaxSecur : Inport  RequirementInfo={} %GIDa_8395a280_2d33_4414_aa2a_4ee33591457b  OutDataTypeStr=single
  Action Port : ActionPort  ActionType=else
  CopyRight2 : Subsystem  Description=|  mask(Copyright Information){none=on}
      | Copyright info block.                                               
      |                                                                     
      | Place copyright information at the top of every subsystem in design.
      mask prompts: none "No parameters"
      mask help: Place copyright information at the top of every subsystem in design.
      mask Display:
      | NxtrConf = 'Nexteer Confidential';
      | 
      | sys = bdroot; %handle for the current model ("system")
      | first = get_param(sys,'Created');
      | if(isempty(first))
      |     first = datestr(now,'yyyy');
      | else
      |     first = first(end-3:end);  %year is last four digits
      | end
      | 
      | last = get_param(sys,'LastModifiedDate');
      | if isempty(last)
      |     last = datestr(now,'yyyy');
      | else
      |     last = last(end-3:end);
      | end
      | 
      | if strcmp(first,last)
      |     fprintf('%s -- Copyright %s Nexteer',NxtrConf,first)
      | else
      |     fprintf('%s -- %s%s- %s Nexteer',NxtrConf,char(169),first,last)
      | end
  TmpVehSpdMaxSecur : Outport
  wires:
  VehSpdMaxSecur/1 -> TmpVehSpdMaxSecur/1

== system CF016A_GmVehSpdArbn/GmVehSpdArbn/GmVehSpdArbnPer1/Calc_VehSpdMaxSecur/Pass_VehSpdMaxSecur1 ==
  VehSpdMaxSecur : Inport  RequirementInfo={} %GIDa_a60723be_98f8_4285_9306_4a7ca9e13402
  Action Port : ActionPort  ActionType=else
  CopyRight2 : Subsystem  Description=|  mask(Copyright Information){none=on}
      | Copyright info block.                                               
      |                                                                     
      | Place copyright information at the top of every subsystem in design.
      mask prompts: none "No parameters"
      mask help: Place copyright information at the top of every subsystem in design.
      mask Display:
      | NxtrConf = 'Nexteer Confidential';
      | 
      | sys = bdroot; %handle for the current model ("system")
      | first = get_param(sys,'Created');
      | if(isempty(first))
      |     first = datestr(now,'yyyy');
      | else
      |     first = first(end-3:end);  %year is last four digits
      | end
      | 
      | last = get_param(sys,'LastModifiedDate');
      | if isempty(last)
      |     last = datestr(now,'yyyy');
      | else
      |     last = last(end-3:end);
      | end
      | 
      | if strcmp(first,last)
      |     fprintf('%s -- Copyright %s Nexteer',NxtrConf,first)
      | else
      |     fprintf('%s -- %s%s- %s Nexteer',NxtrConf,char(169),first,last)
      | end
  TmpVehSpdMaxSecur : Outport
  wires:
  VehSpdMaxSecur/1 -> TmpVehSpdMaxSecur/1

== system CF016A_GmVehSpdArbn/GmVehSpdArbn/GmVehSpdArbnPer1/Calc_VehSpdMaxSecur/Pass_VehSpdMaxSecur2 ==
  VehSpdMaxSecur : Inport  RequirementInfo={} %GIDa_34cfcf7e_ab10_4f2e_bd02_371baa979f8f
  Action Port : ActionPort  ActionType=else
  CopyRight2 : Subsystem  Description=|  mask(Copyright Information){none=on}
      | Copyright info block.                                               
      |                                                                     
      | Place copyright information at the top of every subsystem in design.
      mask prompts: none "No parameters"
      mask help: Place copyright information at the top of every subsystem in design.
      mask Display:
      | NxtrConf = 'Nexteer Confidential';
      | 
      | sys = bdroot; %handle for the current model ("system")
      | first = get_param(sys,'Created');
      | if(isempty(first))
      |     first = datestr(now,'yyyy');
      | else
      |     first = first(end-3:end);  %year is last four digits
      | end
      | 
      | last = get_param(sys,'LastModifiedDate');
      | if isempty(last)
      |     last = datestr(now,'yyyy');
      | else
      |     last = last(end-3:end);
      | end
      | 
      | if strcmp(first,last)
      |     fprintf('%s -- Copyright %s Nexteer',NxtrConf,first)
      | else
      |     fprintf('%s -- %s%s- %s Nexteer',NxtrConf,char(169),first,last)
      | end
  TmpVehSpdMaxSecur : Outport
  wires:
  VehSpdMaxSecur/1 -> TmpVehSpdMaxSecur/1

== system CF016A_GmVehSpdArbn/GmVehSpdArbn/GmVehSpdArbnPer1/Calc_VehSpdMaxSecur/Pass_VehSpdMaxSecur3 ==
  VehSpdMaxSecur : Inport  RequirementInfo={} %GIDa_836c4ab9_430c_4cdb_92f0_24dabab7736b
  Action Port : ActionPort  ActionType=else
  CopyRight2 : Subsystem  Description=|  mask(Copyright Information){none=on}
      | Copyright info block.                                               
      |                                                                     
      | Place copyright information at the top of every subsystem in design.
      mask prompts: none "No parameters"
      mask help: Place copyright information at the top of every subsystem in design.
      mask Display:
      | NxtrConf = 'Nexteer Confidential';
      | 
      | sys = bdroot; %handle for the current model ("system")
      | first = get_param(sys,'Created');
      | if(isempty(first))
      |     first = datestr(now,'yyyy');
      | else
      |     first = first(end-3:end);  %year is last four digits
      | end
      | 
      | last = get_param(sys,'LastModifiedDate');
      | if isempty(last)
      |     last = datestr(now,'yyyy');
      | else
      |     last = last(end-3:end);
      | end
      | 
      | if strcmp(first,last)
      |     fprintf('%s -- Copyright %s Nexteer',NxtrConf,first)
      | else
      |     fprintf('%s -- %s%s- %s Nexteer',NxtrConf,char(169),first,last)
      | end
  TmpVehSpdMaxSecur : Outport
  wires:
  VehSpdMaxSecur/1 -> TmpVehSpdMaxSecur/1

== system CF016A_GmVehSpdArbn/GmVehSpdArbn/GmVehSpdArbnPer1/Calc_VehSpdMinSecurVld/CopyRight2 ==

== system CF016A_GmVehSpdArbn/GmVehSpdArbn/GmVehSpdArbnPer1/Calc_VehSpdMinSecurVld/Get_Min ==
  TmpVehSpdMinSecur : Inport  RequirementInfo={} %GIDa_f93e4fd1_c191_4a73_9f76_15d4e52fe25d
  RiNonDrvnBusChassisExp : Inport  RequirementInfo={} %GIDa_8c898a9e_b3fb_457e_a143_e784d8dd21b6  Port=2
  RiNonDrvnBusHiSpd : Inport  RequirementInfo={} %GIDa_5435686c_ae14_48c3_b024_e80b2dfe6257  Port=3
  Action Port : ActionPort  ActionType=then
  CopyRight2 : Subsystem  Description=|  mask(Copyright Information){none=on}
      | Copyright info block.                                               
      |                                                                     
      | Place copyright information at the top of every subsystem in design.
      mask prompts: none "No parameters"
      mask help: Place copyright information at the top of every subsystem in design.
      mask Display:
      | NxtrConf = 'Nexteer Confidential';
      | 
      | sys = bdroot; %handle for the current model ("system")
      | first = get_param(sys,'Created');
      | if(isempty(first))
      |     first = datestr(now,'yyyy');
      | else
      |     first = first(end-3:end);  %year is last four digits
      | end
      | 
      | last = get_param(sys,'LastModifiedDate');
      | if isempty(last)
      |     last = datestr(now,'yyyy');
      | else
      |     last = last(end-3:end);
      | end
      | 
      | if strcmp(first,last)
      |     fprintf('%s -- Copyright %s Nexteer',NxtrConf,first)
      | else
      |     fprintf('%s -- %s%s- %s Nexteer',NxtrConf,char(169),first,last)
      | end
  Min_f1 : NxtrMin/Min_f32  SFunctionSpec=single y1 = Min_f32(single u1, single u2)
      settings: AttributesFormatString=%<Name>
  Min_f2 : NxtrMin/Min_f32  SFunctionSpec=single y1 = Min_f32(single u1, single u2)
      settings: AttributesFormatString=%<Name>
  TmpMinSpd : Outport
  wires:
  RiNonDrvnBusChassisExp/1 -> Min_f1/2
  TmpVehSpdMinSecur/1 -> Min_f1/1
  Min_f1/1 -> Min_f2/1
  RiNonDrvnBusHiSpd/1 -> Min_f2/2
  Min_f2/1 -> TmpMinSpd/1

== system CF016A_GmVehSpdArbn/GmVehSpdArbn/GmVehSpdArbnPer1/Calc_VehSpdMinSecurVld/Min_LeNonDrvnBusHiSpd_LeNonDrvnBusChassisExp ==
  LeNonDrvnBusHiSpd : Inport  RequirementInfo={} %GIDa_731c71b7_cdf6_4f9d_abaf_45084a573d9f
  LeNonDrvnBusChassisExp : Inport  RequirementInfo={} %GIDa_df06ed12_5996_4272_b401_1f488a4b81b3  Port=2
  Action Port : ActionPort  ActionType=then
  CopyRight2 : Subsystem  Description=|  mask(Copyright Information){none=on}
      | Copyright info block.                                               
      |                                                                     
      | Place copyright information at the top of every subsystem in design.
      mask prompts: none "No parameters"
      mask help: Place copyright information at the top of every subsystem in design.
      mask Display:
      | NxtrConf = 'Nexteer Confidential';
      | 
      | sys = bdroot; %handle for the current model ("system")
      | first = get_param(sys,'Created');
      | if(isempty(first))
      |     first = datestr(now,'yyyy');
      | else
      |     first = first(end-3:end);  %year is last four digits
      | end
      | 
      | last = get_param(sys,'LastModifiedDate');
      | if isempty(last)
      |     last = datestr(now,'yyyy');
      | else
      |     last = last(end-3:end);
      | end
      | 
      | if strcmp(first,last)
      |     fprintf('%s -- Copyright %s Nexteer',NxtrConf,first)
      | else
      |     fprintf('%s -- %s%s- %s Nexteer',NxtrConf,char(169),first,last)
      | end
  Min_f32 : NxtrMin/Min_f32  SFunctionSpec=single y1 = Min_f32(single u1, single u2)
      settings: AttributesFormatString=%<Name>
  TmpMinSpd : Outport
  wires:
  Min_f32/1 -> TmpMinSpd/1
  LeNonDrvnBusHiSpd/1 -> Min_f32/1
  LeNonDrvnBusChassisExp/1 -> Min_f32/2

== system CF016A_GmVehSpdArbn/GmVehSpdArbn/GmVehSpdArbnPer1/Calc_VehSpdMinSecurVld/Pass_VehSpdMinSecur ==
  TmpVehSpdMinSecur : Inport  RequirementInfo={} %GIDa_745b8a7a_b24a_4e8f_b6eb_018455d3aa2c
  Action Port : ActionPort  ActionType=else
  CopyRight2 : Subsystem  Description=|  mask(Copyright Information){none=on}
      | Copyright info block.                                               
      |                                                                     
      | Place copyright information at the top of every subsystem in design.
      mask prompts: none "No parameters"
      mask help: Place copyright information at the top of every subsystem in design.
      mask Display:
      | NxtrConf = 'Nexteer Confidential';
      | 
      | sys = bdroot; %handle for the current model ("system")
      | first = get_param(sys,'Created');
      | if(isempty(first))
      |     first = datestr(now,'yyyy');
      | else
      |     first = first(end-3:end);  %year is last four digits
      | end
      | 
      | last = get_param(sys,'LastModifiedDate');
      | if isempty(last)
      |     last = datestr(now,'yyyy');
      | else
      |     last = last(end-3:end);
      | end
      | 
      | if strcmp(first,last)
      |     fprintf('%s -- Copyright %s Nexteer',NxtrConf,first)
      | else
      |     fprintf('%s -- %s%s- %s Nexteer',NxtrConf,char(169),first,last)
      | end
  TmpMinSpd : Outport
  wires:
  TmpVehSpdMinSecur/1 -> TmpMinSpd/1

== system CF016A_GmVehSpdArbn/GmVehSpdArbn/GmVehSpdArbnPer1/Calc_VehSpdMinSecurVld/Set_VehSpdMinSecur_Max ==
  TmpVehSpdMinSecur : Inport  RequirementInfo={} %GIDa_3ff90c3f_2eb6_4f81_90c1_1df8352fc446
  Action Port : ActionPort  ActionType=else
  CopyRight2 : Subsystem  Description=|  mask(Copyright Information){none=on}
      | Copyright info block.                                               
      |                                                                     
      | Place copyright information at the top of every subsystem in design.
      mask prompts: none "No parameters"
      mask help: Place copyright information at the top of every subsystem in design.
      mask Display:
      | NxtrConf = 'Nexteer Confidential';
      | 
      | sys = bdroot; %handle for the current model ("system")
      | first = get_param(sys,'Created');
      | if(isempty(first))
      |     first = datestr(now,'yyyy');
      | else
      |     first = first(end-3:end);  %year is last four digits
      | end
      | 
      | last = get_param(sys,'LastModifiedDate');
      | if isempty(last)
      |     last = datestr(now,'yyyy');
      | else
      |     last = last(end-3:end);
      | end
      | 
      | if strcmp(first,last)
      |     fprintf('%s -- Copyright %s Nexteer',NxtrConf,first)
      | else
      |     fprintf('%s -- %s%s- %s Nexteer',NxtrConf,char(169),first,last)
      | end
  TmpMinSpd : Outport
  wires:
  TmpVehSpdMinSecur/1 -> TmpMinSpd/1

== system CF016A_GmVehSpdArbn/GmVehSpdArbn/GmVehSpdArbnPer1/LeDrvnVld/CopyRight2 ==
